simulink model "BUCKBO_1"  (R2020b)
settings: Solver=VariableStepAuto  StartTime=0.0  StopTime=1  RelTol=1e-3
libraries: spsCurrentMeasurementLib x6, spsVoltageMeasurementLib x4, spsSeriesRLCBranchLib x3, spsDCVoltageSourceLib x1, spsDiodeLib x1, spsMosfetLib x1, simulink x1, dspstat3 x1, spspowerguiLib x1
settings Model: Creator=HeriRakouth  LastModifiedBy=HeriRakouth
settings DebuggingCC: SFMachineParentedDataDiag=error

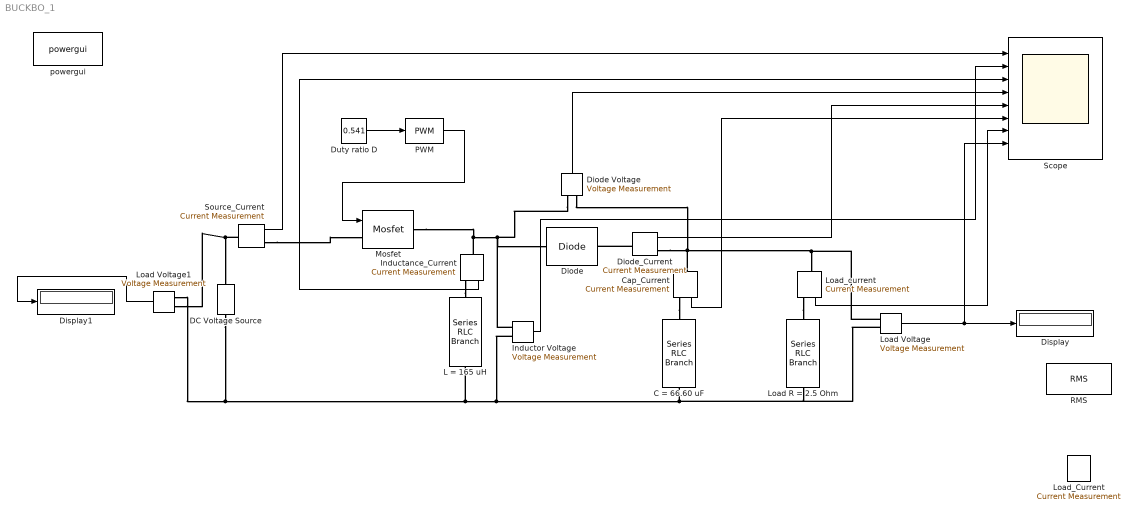
== system BUCKBO_1 ==
  C = 66.60 uF : spsSeriesRLCBranchLib/Series RLC Branch  LConnTagsString=__new0  RConnTagsString=__new0  BranchType=C  Resistance=0  Inductance=0  SetiL0=off  InitialCurrent=0  Capacitance=66.60e-6  Setx0=off  InitialVoltage=0  Measurements=None
  Cap_Current : spsCurrentMeasurementLib/Current Measurement  PhasorSimulation=off  OutputType=Complex  PSBequivalent=0
  DC Voltage Source : spsDCVoltageSourceLib/DC Voltage Source  Amplitude=40  Measurements=None
  Diode : spsDiodeLib/Diode  Ron=0.001  Lon=0  Vf=0.0001  IC=0  UseSnubber=0  Rs=1e6  Cs=0  Measurements=off
  Diode Voltage : spsVoltageMeasurementLib/Voltage Measurement  PhasorSimulation=off  OutputType=Complex  PSBequivalent=0
  Diode_Current : spsCurrentMeasurementLib/Current Measurement  PhasorSimulation=off  OutputType=Complex  PSBequivalent=0
  Display : Display
  Display1 : Display
  Duty ratio D : Constant  Value=0.541
  Inductance_Current : spsCurrentMeasurementLib/Current Measurement  PhasorSimulation=off  OutputType=Complex  PSBequivalent=0
  Inductor Voltage : spsVoltageMeasurementLib/Voltage Measurement  PhasorSimulation=off  OutputType=Complex  PSBequivalent=0
  L = 165 uH : spsSeriesRLCBranchLib/Series RLC Branch  LConnTagsString=__new0  RConnTagsString=__new0  BranchType=L  Resistance=0  Inductance=165e-6  SetiL0=off  InitialCurrent=0  Capacitance=0  Setx0=off  InitialVoltage=0  Measurements=None
  Load R = 2.5 Ohm : spsSeriesRLCBranchLib/Series RLC Branch  LConnTagsString=__new0  RConnTagsString=__new0  BranchType=R  Resistance=2.5  Inductance=0  SetiL0=off  InitialCurrent=0  Capacitance=0  Setx0=off  InitialVoltage=0  Measurements=None
  Load Voltage : spsVoltageMeasurementLib/Voltage Measurement  PhasorSimulation=off  OutputType=Complex  PSBequivalent=0
  Load Voltage1 : spsVoltageMeasurementLib/Voltage Measurement  PhasorSimulation=off  OutputType=Complex  PSBequivalent=0
  Load_Current : spsCurrentMeasurementLib/Current Measurement  PhasorSimulation=off  OutputType=Complex  PSBequivalent=0
  Load_current : spsCurrentMeasurementLib/Current Measurement  PhasorSimulation=off  OutputType=Complex  PSBequivalent=0
  Mosfet : spsMosfetLib/Mosfet  Ron=0.0001  Lon=0  Rd=0.0001  Vfd=0.0001  IC=0  Rs=1e5  Cs=0  Measurements=off
  PWM : simulink/Discontinuities/PWM  DisableCoverage=on  Period=4e-5  DisallowZeroDutyCycle=off  RunAtFixedTimeIntervals=off  SampleTime=0.1
  RMS : dspstat3/RMS  run=off  directionMode=Each column  dimension=1  InputProcessing=Columns as channels (frame based)  reset_popup=None
  Scope : Scope  NumInputPorts=8
  Source_Current : spsCurrentMeasurementLib/Current Measurement  PhasorSimulation=off  OutputType=Complex  PSBequivalent=0
  powergui : spspowerguiLib/powergui  Priority=1  SimulationMode=Continuous  SampleTime=50e-6  frequency=60  Iterations=50  frequencyindice=0  Pbase=100e6  ErrMax=1e-4  UnitsV=kV  UnitsW=MW  buscounter=0  FunctionMessages=off  echomessages=off  EnableUseOfTLC=off  CurrentSourceSwitches=off  DisableSnubberDevices=off  DisableRonSwitches=off  DisableVfSwitches=off  DisplayEquations=off  AutomaticDiscreteSolvers=off  SolverType=Tustin/Backward Euler (TBE)  Interpol=off  ExternalGateDelay=off  methode=off  Ts=100  x0status=blocks  SPID=on  SwTol=0  HookPort=off  NonlinearTolerance=1e-4  nMaxIteration=100  ContinueOnMaxIteration=off  RestoreLinks=warning  ResistiveCurrentMeasurement=off  Frange=[0:2:500]  Ylog=off  Xlog=on  ShowGrid=off  save=off  variable=ZData  structure=0  ZoomFFT=off  StartTime=0.0  cycles=1  DisplayStyle=1  fundamental=60  FreqAxis=off  MaxFrequency=1000  frequencyindicesteady=1  RmsSteady=1  display=off
  wires:
  Source_Current/1 -> Scope/1
  Inductance_Current/1 -> Scope/3
  Inductor Voltage/1 -> Scope/2
  Diode Voltage/1 -> Scope/4
  Diode_Current/1 -> Scope/5
  Cap_Current/1 -> Scope/6
  Load_current/1 -> Scope/7
  Load Voltage/1 -> Display/1, Scope/8
  Duty ratio D/1 -> PWM/1
  PWM/1 -> Mosfet/1
  Load Voltage1/1 -> Display1/1
  connections:
  Source_Current/LConn1 -- Load Voltage1/LConn1 -- DC Voltage Source/RConn1
  Mosfet/RConn1 -- Inductance_Current/LConn1 -- Diode Voltage/LConn1 -- Diode/RConn1 -- Inductor Voltage/LConn1
  Inductance_Current/RConn1 -- L = 165 uH/LConn1
  DC Voltage Source/LConn1 -- Load Voltage1/LConn2 -- Inductor Voltage/LConn2 -- Load Voltage/LConn2 -- Load R = 2.5 Ohm/RConn1 -- C = 66.60 uF/RConn1 -- L = 165 uH/RConn1
  Cap_Current/RConn1 -- C = 66.60 uF/LConn1
  Diode_Current/LConn1 -- Diode/LConn1
  Load_current/RConn1 -- Load R = 2.5 Ohm/LConn1
  Diode_Current/RConn1 -- Diode Voltage/LConn2 -- Load Voltage/LConn1 -- Load_current/LConn1 -- Cap_Current/LConn1
  Source_Current/RConn1 -- Mosfet/LConn1
